simulink model "Problem_1"  (R2020a)
settings: Solver=VariableStepAuto  StartTime=0.0  StopTime=10.0  RelTol=1e-3
settings Model: Creator=user  LastModifiedBy=user

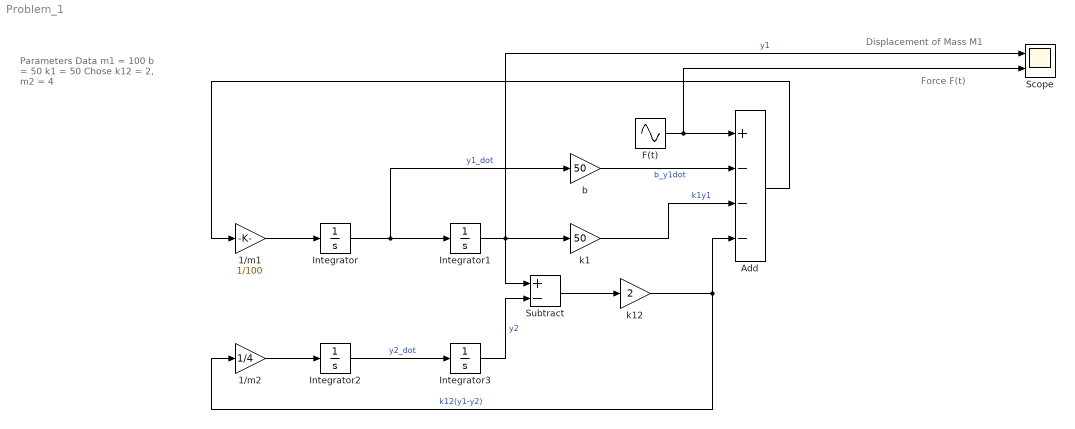
== system Problem_1 ==
  note: Parameters Data
      | m1 = 100
      | b = 50
      | k1 = 50
      | Chose k12 = 2, m2 = 4
  note: Force F(t)
  note: Displacement of Mass M1
  1/m1 : Gain  Gain=1/100
  1/m2 : Gain  Gain=1/4
  Add : Sum  Inputs=+---
  F(t) : Sin  Amplitude=2  Frequency=10  SampleTime=0
  Integrator{,1..3} (4 alike) : Integrator
  Scope : Scope  NumInputPorts=2
  Subtract : Sum  Inputs=+-
  b : Gain  Gain=50
  k1 : Gain  Gain=50
  k12 : Gain  Gain=2
  wires:
  Integrator/1 -> b/1, Integrator1/1  "y1_dot"
  Integrator2/1 -> Integrator3/1  "y2_dot"
  Integrator1/1 -> Scope/1, k1/1, Subtract/1  "y1"
  Integrator3/1 -> Subtract/2  "y2"
  F(t)/1 -> Scope/2, Add/1
  b/1 -> Add/2  "b_y1dot"
  k1/1 -> Add/3  "k1y1"
  Subtract/1 -> k12/1
  k12/1 -> 1/m2/1, Add/4  "k12(y1-y2)"
  1/m1/1 -> Integrator/1
  Add/1 -> 1/m1/1
  1/m2/1 -> Integrator2/1
